simulink model "sampleModel1482"  (R2023a)
settings: Solver=VariableStepAuto  StartTime=0.0  StopTime=10.0  RelTol=1e-3
libraries: hdlsllib x4, simulink x2
settings Model: Creator=user1  LastModifiedBy=user1

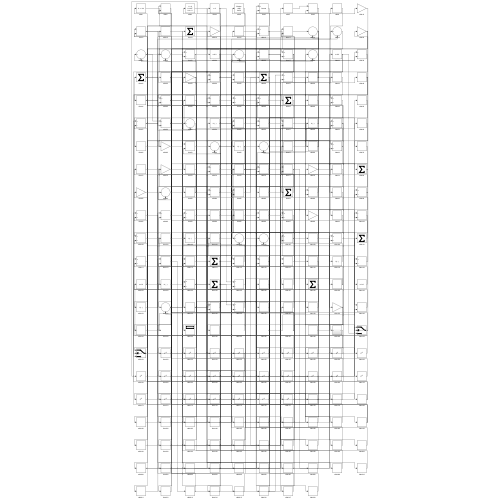
[thumbnail: Simulink's stored preview of the top-level diagram]
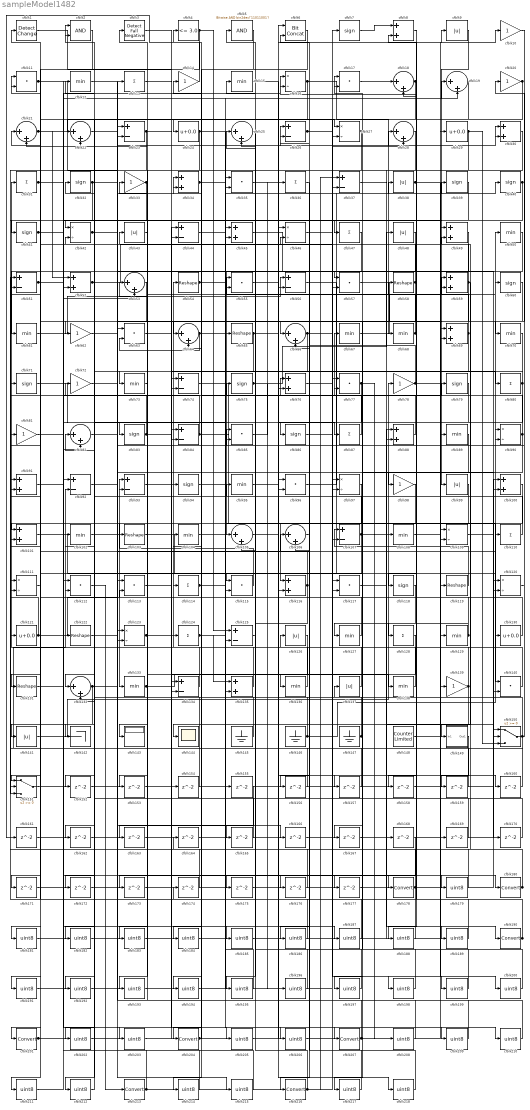
== system sampleModel1482 ==
  cfblk1 : simulink/Logic and Bit Operations/Detect Change  vinit=0  OutDataTypeStr=boolean
      settings: LibrarySourceBlock=|
      | hdlsllib/Logic and Bit
      | Operations/Detect
      | Change
  cfblk{10,14,20,33,62,72,78,81,98,139} (10 alike) : Gain
  cfblk{8,30,34,45,49,52,59,69,76,88,91,100..101,116,135} (15 alike) : Sum
  cfblk{12,15,50,61,67..68,70,73,89,95,102,104,108,127,129,133,136,138} (18 alike) : MinMax
  cfblk{54,58,65,103,119,122,131} (7 alike) : Reshape
  cfblk{18..19,21..22,25,28,53,64,66,82,105..106,132} (13 alike) : Sum  Inputs=|++
  cfblk{23,26,37,44,51,56,74,84,92..93,107,125,134} (13 alike) : Sum  Inputs=+-
  cfblk{16,27,42,46,90,97,109,111,120,123} (10 alike) : Product  Inputs=*/  RndMeth=Zero  SaturateOnIntegerOverflow=on
  cfblk{11,17,35,55,57,63,77,85,96,112..113,115,117,140} (14 alike) : DotProduct  OutDataTypeStr=Inherit: Inherit via internal rule
  cfblk{13,31,36,47,80,87,110,114,124,128} (10 alike) : Sum  Inputs=+
  cfblk{7,32,39..41,60,71,75,79,83,86,94,118} (13 alike) : Signum
  cfblk{24,29,121,130} (4 alike) : Bias  Bias=0.0  SaturateOnIntegerOverflow=off
  cfblk{9,38,43,48,99,126,137,141} (8 alike) : Abs  SaturateOnIntegerOverflow=off
  cfblk142 : Terminator
  cfblk143 : Display
  cfblk144 : Scope
  cfblk145 : Ground
  cfblk146 : Ground
  cfblk147 : Ground
  cfblk148 : hdlsllib/Sources/Counter Limited  uplimit=7  tsamp=-1
  cfblk149 : Subsystem
      settings: LibrarySourceBlock=|
      | hdlsllib/Ports &
      | Subsystems/Subsystem
  cfblk150 : Switch  SaturateOnIntegerOverflow=off  InputSameDT=off
  cfblk151 : Switch  SaturateOnIntegerOverflow=off  InputSameDT=off
  cfblk{152..177} (26 alike) : Delay  SampleTime=1
  cfblk{178,180,190,201,204,207,213,216} (8 alike) : DataTypeConversion  SaturateOnIntegerOverflow=off  RndMeth=Floor
  cfblk{179,181..189,191..200,202..203,205..206,208..212,214..215,217..218} (33 alike) : DataTypeConversion  OutDataTypeStr=uint8  SaturateOnIntegerOverflow=off  RndMeth=Floor
  cfblk2 : Logic  AllPortsSameDT=off  OutDataTypeStr=boolean
  cfblk3 : hdlsllib/Logic and Bit Operations/Detect Fall Negative  vinit=0  OutDataTypeStr=boolean
  cfblk4 : hdlsllib/Logic and Bit Operations/Compare To Constant  relop=<=  const=3.0  OutDataTypeStr=boolean
  cfblk5 : simulink/Logic and Bit Operations/Bitwise Operator  logicop=AND  UseBitMask=on  BitMask=bin2dec('11011001')  BitMaskRealWorld=Stored Integer
      settings: LibrarySourceBlock=|
      | hdlsllib/Logic and Bit
      | Operations/Bitwise
      | Operator
  cfblk6 : hdlsllib/Logic and Bit Operations/Bit Concat  numInputs=2
  wires:
  cfblk121/1 -> cfblk31/1, cfblk23/1
  cfblk26/1 -> cfblk28/2, cfblk160/1
  cfblk85/1 -> cfblk36/1
  cfblk135/1 -> cfblk54/1
  cfblk141/1 -> cfblk78/1
  cfblk17/1 -> cfblk18/1
  cfblk117/1 -> cfblk190/1
  cfblk146/1 -> cfblk50/1, cfblk72/1
  cfblk6/1 -> cfblk204/1
  cfblk116/1 -> cfblk132/1, cfblk71/1
  cfblk28/1 -> cfblk88/2
  cfblk97/1 -> cfblk201/1
  cfblk103/1 -> cfblk115/1
  cfblk150/1 -> cfblk92/2, cfblk20/1, cfblk76/1
  cfblk38/1 -> cfblk16/1, cfblk200/1
  cfblk110/1 -> cfblk32/1
  cfblk107/1 -> cfblk93/1, cfblk208/1, cfblk211/1
  cfblk9/1 -> cfblk99/1
  cfblk69/1 -> cfblk5/1, cfblk192/1
  cfblk11/1 -> cfblk63/1, cfblk203/1
  cfblk96/1 -> cfblk40/1
  cfblk51/1 -> cfblk82/2, cfblk19/1
  cfblk21/1 -> cfblk27/1, cfblk52/1
  cfblk138/1 -> cfblk81/1
  cfblk106/1 -> cfblk216/1
  cfblk133/1 -> cfblk138/1, cfblk209/1
  cfblk43/1 -> cfblk83/1
  cfblk67/1 -> cfblk59/1
  cfblk87/1 -> cfblk14/1
  cfblk73/1 -> cfblk33/1
  cfblk131/1 -> cfblk79/1
  cfblk132/1 -> cfblk141/1, cfblk110/1, cfblk28/1
  cfblk13/1 -> cfblk27/2
  cfblk16/1 -> cfblk68/1, cfblk101/1
  cfblk72/1 -> cfblk13/1
  cfblk115/1 -> cfblk93/2
  cfblk48/1 -> cfblk105/1
  cfblk61/1 -> cfblk56/1
  cfblk99/1 -> cfblk116/1
  cfblk112/1 -> cfblk213/1
  cfblk129/1 -> cfblk128/1, cfblk101/2
  cfblk78/1 -> cfblk10/1, cfblk42/2
  cfblk102/1 -> cfblk133/1
  cfblk124/1 -> cfblk104/1, cfblk90/2, cfblk135/1, cfblk214/1
  cfblk31/1 -> cfblk16/2, cfblk53/2
  cfblk148/1 -> cfblk29/1
  cfblk151/1 -> cfblk96/1
  cfblk18/1 -> cfblk152/1, cfblk202/1
  cfblk80/1 -> cfblk73/1, cfblk172/1
  cfblk74/1 -> cfblk140/1
  cfblk27/1 -> cfblk142/1, cfblk103/1
  cfblk66/1 -> cfblk153/1, cfblk199/1
  cfblk84/1 -> cfblk119/1, cfblk2/2
  cfblk137/1 -> cfblk55/1
  cfblk62/1 -> cfblk69/1
  cfblk10/1 -> cfblk70/1
  cfblk113/1 -> cfblk207/1
  cfblk92/1 -> cfblk26/1
  cfblk140/1 -> cfblk95/1
  cfblk39/1 -> cfblk65/1
  cfblk101/1 -> cfblk130/1
  cfblk145/1 -> cfblk114/1
  cfblk82/1 -> cfblk100/2
  cfblk50/1 -> cfblk61/1
  cfblk128/1 -> cfblk143/1
  cfblk23/1 -> cfblk52/2, cfblk165/1
  cfblk54/1 -> cfblk39/1, cfblk107/2
  cfblk64/1 -> cfblk63/2, cfblk19/2, cfblk179/1
  cfblk65/1 -> cfblk125/2, cfblk218/1
  cfblk40/1 -> cfblk84/2, cfblk62/1
  cfblk59/1 -> cfblk127/1, cfblk8/2, cfblk149/1(In1)
  cfblk111/1 -> cfblk151/1
  cfblk83/1 -> cfblk98/1, cfblk11/1
  cfblk71/1 -> cfblk124/1
  cfblk56/1 -> cfblk129/1
  cfblk88/1 -> cfblk15/1
  cfblk108/1 -> cfblk139/1
  cfblk127/1 -> cfblk34/1
  cfblk68/1 -> cfblk66/1, cfblk21/2
  cfblk52/1 -> cfblk7/1, cfblk166/1
  cfblk5/1 -> cfblk64/1
  cfblk41/1 -> cfblk49/1, cfblk175/1
  cfblk136/1 -> cfblk2/1
  cfblk35/1 -> cfblk180/1
  cfblk4/1 -> cfblk125/1, cfblk181/1
  cfblk134/1 -> cfblk111/2
  cfblk3/1 -> cfblk178/1
  cfblk42/1 -> cfblk56/2, cfblk34/2
  cfblk95/1 -> cfblk9/1
  cfblk125/1 -> cfblk75/1
  cfblk119/1 -> cfblk17/1
  cfblk2/1 -> cfblk131/1
  cfblk55/1 -> cfblk57/1
  cfblk120/1 -> cfblk90/1
  cfblk63/1 -> cfblk80/1
  cfblk33/1 -> cfblk42/1, cfblk173/1
  cfblk130/1 -> cfblk102/1
  cfblk90/1 -> cfblk67/1, cfblk118/1
  cfblk15/1 -> cfblk87/1
  cfblk76/1 -> cfblk57/2
  cfblk57/1 -> cfblk89/1
  cfblk114/1 -> cfblk30/1, cfblk144/1
  cfblk24/1 -> cfblk136/1, cfblk162/1, cfblk212/1
  cfblk147/1 -> cfblk64/2, cfblk53/1
  cfblk19/1 -> cfblk41/1
  cfblk104/1 -> cfblk59/2
  cfblk29/1 -> cfblk151/3, cfblk150/3, cfblk182/1
  cfblk139/1 -> cfblk107/1, cfblk194/1, cfblk197/1
  cfblk7/1 -> cfblk8/1
  cfblk100/1 -> cfblk123/2
  cfblk30/1 -> cfblk105/2
  cfblk122/1 -> cfblk85/1
  cfblk20/1 -> cfblk24/1, cfblk23/2
  cfblk86/1 -> cfblk60/1
  cfblk58/1 -> cfblk21/1, cfblk86/1, cfblk11/2
  cfblk81/1 -> cfblk85/2
  cfblk123/1 -> cfblk74/2, cfblk135/2
  cfblk45/1 -> cfblk120/2
  cfblk77/1 -> cfblk115/2, cfblk108/1
  cfblk75/1 -> cfblk48/1, cfblk177/1, cfblk196/1
  cfblk32/1 -> cfblk151/2, cfblk215/1
  cfblk94/1 -> cfblk38/1
  cfblk1/1 -> cfblk44/2
  cfblk37/1 -> cfblk150/2
  cfblk34/1 -> cfblk47/1, cfblk30/2
  cfblk98/1 -> cfblk134/2
  cfblk153/1 -> cfblk100/1
  cfblk93/1 -> cfblk154/1
  cfblk154/1 -> cfblk82/1
  cfblk47/1 -> cfblk156/1
  cfblk156/1 -> cfblk111/1
  cfblk105/1 -> cfblk157/1
  cfblk157/1 -> cfblk84/1
  cfblk8/1 -> cfblk158/1
  cfblk158/1 -> cfblk18/2
  cfblk149/1(Out1) -> cfblk159/1
  cfblk159/1 -> cfblk51/2
  cfblk160/1 -> cfblk92/1
  cfblk14/1 -> cfblk161/1
  cfblk161/1 -> cfblk88/1
  cfblk162/1 -> cfblk120/1
  cfblk79/1 -> cfblk163/1
  cfblk163/1 -> cfblk45/2
  cfblk164/1 -> cfblk150/1
  cfblk165/1 -> cfblk123/1
  cfblk166/1 -> cfblk66/2
  cfblk89/1 -> cfblk167/1
  cfblk169/1 -> cfblk17/2
  cfblk109/1 -> cfblk170/1
  cfblk170/1 -> cfblk132/2
  cfblk60/1 -> cfblk171/1
  cfblk171/1 -> cfblk96/2
  cfblk172/1 -> cfblk134/1
  cfblk173/1 -> cfblk69/2
  cfblk174/1 -> cfblk1/1
  cfblk175/1 -> cfblk116/2
  cfblk49/1 -> cfblk176/1
  cfblk176/1 -> cfblk74/1
  cfblk177/1 -> cfblk140/2
  cfblk178/1 -> cfblk174/1, cfblk121/1
  cfblk179/1 -> cfblk3/1
  cfblk180/1 -> cfblk49/2, cfblk51/1
  cfblk181/1 -> cfblk35/1
  cfblk182/1 -> cfblk35/2
  cfblk168/1 -> cfblk183/1
  cfblk183/1 -> cfblk44/1
  cfblk126/1 -> cfblk184/1
  cfblk184/1 -> cfblk168/1
  cfblk12/1 -> cfblk185/1
  cfblk185/1 -> cfblk109/1
  cfblk36/1 -> cfblk186/1
  cfblk186/1 -> cfblk12/1
  cfblk91/1 -> cfblk187/1
  cfblk187/1 -> cfblk43/1
  cfblk70/1 -> cfblk188/1
  cfblk188/1 -> cfblk91/1
  cfblk167/1 -> cfblk189/1
  cfblk189/1 -> cfblk91/2
  cfblk190/1 -> cfblk58/1, cfblk26/2, cfblk137/1
  cfblk53/1 -> cfblk191/1
  cfblk191/1 -> cfblk117/1
  cfblk192/1 -> cfblk117/2
  cfblk155/1 -> cfblk193/1
  cfblk193/1 -> cfblk77/1
  cfblk194/1 -> cfblk155/1
  cfblk25/1 -> cfblk195/1
  cfblk195/1 -> cfblk45/1
  cfblk196/1 -> cfblk25/1
  cfblk197/1 -> cfblk25/2
  cfblk46/1 -> cfblk198/1
  cfblk198/1 -> cfblk77/2
  cfblk199/1 -> cfblk46/1
  cfblk200/1 -> cfblk46/2
  cfblk201/1 -> cfblk76/2, cfblk94/1
  cfblk202/1 -> cfblk97/1
  cfblk203/1 -> cfblk97/2
  cfblk204/1 -> cfblk109/2, cfblk4/1
  cfblk152/1 -> cfblk205/1
  cfblk205/1 -> cfblk6/1
  cfblk44/1 -> cfblk206/1
  cfblk206/1 -> cfblk6/2
  cfblk207/1 -> cfblk169/1, cfblk126/1
  cfblk208/1 -> cfblk113/1
  cfblk209/1 -> cfblk113/2
  cfblk22/1 -> cfblk210/1
  cfblk210/1 -> cfblk164/1
  cfblk211/1 -> cfblk22/1
  cfblk212/1 -> cfblk22/2
  cfblk213/1 -> cfblk122/1, cfblk37/2
  cfblk214/1 -> cfblk112/1
  cfblk215/1 -> cfblk112/2
  cfblk216/1 -> cfblk55/2, cfblk37/1
  cfblk118/1 -> cfblk217/1
  cfblk217/1 -> cfblk106/1
  cfblk218/1 -> cfblk106/2

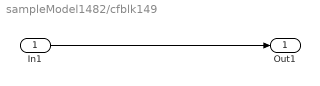
== system sampleModel1482/cfblk149 ==
  In1 : Inport
  Out1 : Outport
  wires:
  In1/1 -> Out1/1
